simulink model "esercizio1_punto1"  (Simulink 7.6)
settings: Solver=ode45  StartTime=0.0  StopTime=10  MaxStep=.1  RelTol=1e-3  AbsTol=1e-3
values from neighbouring files (symbols this model uses):
  den = 1    [ASS1_SIS.M]    (also in ASS_APPR.M; ASS_SIS.M; MYFBODE.M = b; MYNYQ.M = b)
  den_appr = 1    [ASS_APPR.M]    (also in ASS_SIS.M)
  num = 0    [ASS1_SIS.M]    (also in ASS_SIS.M; MYFBODE.M = a; MYNYQ.M = a; nyquistnew.m = a)
  num_appr = 0    [ASS_APPR.M]
  T = 0    [ASS1_SIS.M]    (also in ASS_APPR.M = 0; end; ASS_SIS.M; MYFBODE.M = rit)
  T_appr = 0    [ASS_APPR.M]    (also in ASS_SIS.M = 0; end)
undefined symbols (not defined in the file or in its folder): ht, sfunyst, stt
settings Model: Creator=Ins  LastModifiedBy=Ins  ExtModeTrigMode=oneshot  ExtModeArmWhenConnect=off
settings DataIOCC: LimitDataPoints=off  SaveOutput=off  SaveTime=off  SignalLoggingName=sigsOut
settings OptimizationCC: BooleanDataType=off
settings DebuggingCC: SaveWithParameterizedLinksMsg=none  SignalResolutionControl=TryResolveAllWithWarning  SolverPrmCheckMsg=none  MultiTaskDSMMsg=warning  MultiTaskCondExecSysMsg=none  StrictBusMsg=None
settings HardwareCC: TargetUnknown=on
settings RTWCC: IncludeERTFirstTime=on

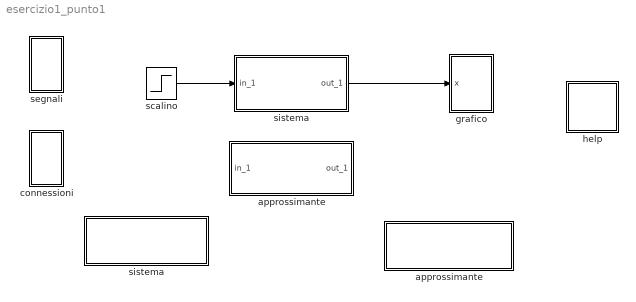
== system esercizio1_punto1 ==
  approssimante : Subsystem
      mask Display: disp('approssimante')
  "approssimante " : Subsystem
      settings: OpenFcn=blocca
      mask Display: disp('approssimante')
  connessioni : Subsystem
  grafico : Subsystem  mask(Storage scope.){npts =2000,  color ='b-/r-/c-./w:/m*/ro/b+'}
      mask prompts: npts  "Initial Time Range:";  color  "Initial y-min:"
      mask help:
      | Storage scope using MATLAB graph window.
      | Enter plotting ranges and line type.
      mask init:
      | ax = [0, @1, @2, @3]; dt=-1;
      mask Help: This block uses a MATLAB figure window to plot the input signal.  The graph limits are automatically scaled to the min and max values of the signal stored in the scope's signal buffer.  Line type must be in quotes.  See the M-file sfunyst.m.
      mask Display: plot(0,0,100,100,[83,76,63,52,42,38,28,16,11,84,11,11,11,90,90,11],[75,58,47,54,72,80,84,74,65,65,65,90,40,40,90,90])
  help : Subsystem
      mask Display: disp('?')
  scalino : Step  Time=0
  segnali : Subsystem
  sistema : Subsystem
      mask Display: disp('sistema')
  "sistema " : Subsystem
      settings: OpenFcn=blocca
      mask Display: disp('sistema')
  wires:
  "sistema "/1(out_1) -> grafico/1(x)
  scalino/1 -> "sistema "/1(in_1)

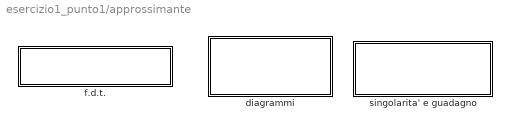
== system esercizio1_punto1/approssimante ==
  diagrammi : Subsystem
      mask Display: disp('diagrammi\n  \n (Bode e Nyquist)')
  f.d.t. : Subsystem
      settings: OpenFcn=ass_appr
      mask Type: assegnamento f.d.t.
      mask Display: disp('assegnamento f.d.t.')
  singolarita' e guadagno : Subsystem
      settings: OpenFcn=sing_app
      mask Type: singolarita' della f.d.t.
      mask Display: disp('singolarità,\n guadagno e ritardo')

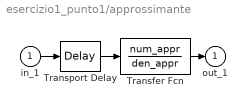
== system esercizio1_punto1/approssimante  ==
  in_1 : Inport
  Transfer Fcn : TransferFcn  Numerator=num_appr  Denominator=den_appr
  Transport Delay : TransportDelay  DelayTime=T_appr
  out_1 : Outport
  wires:
  Transport Delay/1 -> Transfer Fcn/1
  in_1/1 -> Transport Delay/1
  Transfer Fcn/1 -> out_1/1

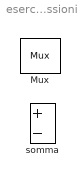
== system esercizio1_punto1/connessioni ==
  Mux : Mux  Inputs=2
  somma : Sum  Inputs=+-  SaturateOnIntegerOverflow=on  InputSameDT=on  OutDataTypeStr=Inherit: Same as first input

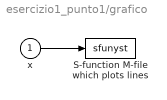
== system esercizio1_punto1/grafico ==
  x : Inport
  "S-function M-file which plots lines " : S-Function  LoadFcn=sfunyst([],[],[],'LoadBlock')  FunctionName=sfunyst  Parameters=ax, color, npts, dt  EnableBusSupport=off
      settings: CopyFcn=sfunyst([],[],[],'CopyBlock')  DeleteFcn=sfunyst([],[],[],'DeleteBlock')
  wires:
  x/1 -> "S-function M-file which plots lines "/1

== system esercizio1_punto1/help ==
  note: - il calcolo delle singolarità (poli e zeri), del guadagno e del ritardo della f.d.t.
  note: - l'inserimento della funzione di trasferimento
  note: - l'ottenimento dei diagrammi di Bode e di Nyquist
  note: i blocchi con l'ombreggiatura consentono

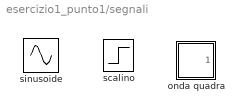
== system esercizio1_punto1/segnali ==
  onda quadra : Subsystem  mask(Pulse Generator){Ts=2,  du=1,  ht=1,  stt=0}
      mask prompts: Ts "Pulse period (secs):";  du "Pulse width:";  ht "Pulse height:";  stt "Pulse start time:"
      mask help: Pulse Generator.
      mask init:
      | ini=ones(length(ht),1); st1=rem(stt,Ts); st2=rem(stt+du,Ts);if(Ts<=1.2*du),ini=zeros(length(ht),1);end;
      mask Help: Pulse generator which ensures pulse\ntransitions are hit. Provides a vector of pulses when the height is entered as a vector.\nUnmask to see how it works.
      mask Display: plot(0,0,100,100,[90,75,75,60,60,35,35,20,20,10],[20,20,80,80,20,20,80,80,20,20])
  scalino : Step  Time=0
  sinusoide : Sin

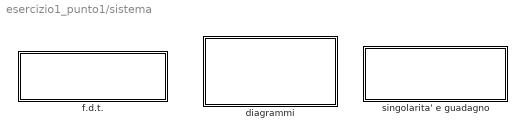
== system esercizio1_punto1/sistema ==
  diagrammi : Subsystem
      mask Display: disp('diagrammi\n  \n (Bode e Nyquist)')
  f.d.t. : Subsystem
      settings: OpenFcn=ass_sis
      mask Type: assegnamento f.d.t.
      mask Display: disp('assegnamento f.d.t.')
  singolarita' e guadagno : Subsystem
      settings: OpenFcn=sing_s
      mask Type: singolarita' della f.d.t.
      mask Display: disp('singolarità,\n guadagno e ritardo')

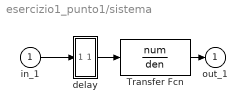
== system esercizio1_punto1/sistema  ==
  in_1 : Inport
  Transfer Fcn : TransferFcn  Numerator=num  Denominator=den
  delay : Subsystem
  out_1 : Outport
  wires:
  delay/1(out_1) -> Transfer Fcn/1
  in_1/1 -> delay/1(in_1)
  Transfer Fcn/1 -> out_1/1

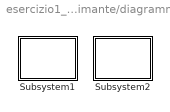
== system esercizio1_punto1/approssimante/diagrammi ==
  Subsystem1 : Subsystem
      settings: OpenFcn=nyq_appr
      mask Display: disp('Nyquist')
  Subsystem2 : Subsystem
      settings: OpenFcn=bode_app
      mask Display: disp('Bode')

== system esercizio1_punto1/approssimante/f.d.t. ==
  note: assegna

== system esercizio1_punto1/approssimante/singolarita' e guadagno ==
  note: assegna

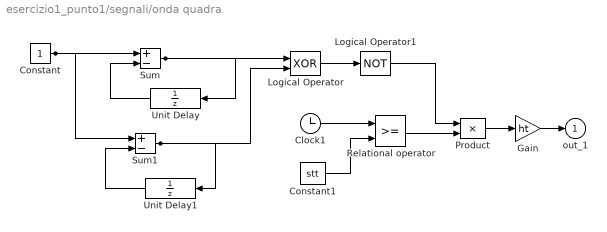
== system esercizio1_punto1/segnali/onda quadra ==
  Clock1 : Clock
      settings: Decimation=10
  Constant : Constant
  Constant1 : Constant  Value=stt
  Gain : Gain  Gain=ht  SaturateOnIntegerOverflow=on  OutDataTypeStr=Inherit: Same as input  ParamDataTypeStr=Inherit: Same as input
  Logical Operator : Logic  Operator=XOR
  Logical Operator1 : Logic  Operator=NOT  Inputs=1
  Product : Product  SaturateOnIntegerOverflow=on  InputSameDT=on  OutDataTypeStr=Inherit: Same as first input
  Relational operator : RelationalOperator  InputSameDT=on
  Sum : Sum  Inputs=+-  SaturateOnIntegerOverflow=on  InputSameDT=on  OutDataTypeStr=Inherit: Same as first input
  Sum1 : Sum  Inputs=+-  SaturateOnIntegerOverflow=on  InputSameDT=on  OutDataTypeStr=Inherit: Same as first input
  Unit Delay : UnitDelay  SampleTime=[Ts,st1]
  Unit Delay1 : UnitDelay  X0=ini  SampleTime=[Ts,st2]
  out_1 : Outport
  wires:
  Logical Operator1/1 -> Product/1
  Logical Operator/1 -> Logical Operator1/1
  Constant1/1 -> Relational operator/2
  Gain/1 -> out_1/1
  Product/1 -> Gain/1
  Relational operator/1 -> Product/2
  Clock1/1 -> Relational operator/1
  Unit Delay/1 -> Sum/2
  Unit Delay1/1 -> Sum1/2
  Constant/1 -> Sum/1, Sum1/1
  Sum/1 -> Unit Delay/1, Logical Operator/1
  Sum1/1 -> Unit Delay1/1, Logical Operator/2

== system esercizio1_punto1/sistema/diagrammi ==
  Bode : Subsystem
      settings: OpenFcn=bode_sis
      mask Display: disp('Bode')
  Nyquist : Subsystem
      settings: OpenFcn=nyq_sis
      mask Display: disp('Nyquist')

== system esercizio1_punto1/sistema/f.d.t. ==
  note: assegna

== system esercizio1_punto1/sistema/singolarita' e guadagno ==
  note: assegna

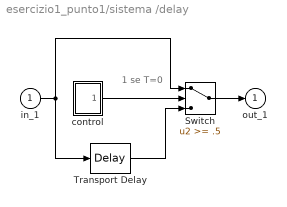
== system esercizio1_punto1/sistema /delay ==
  note: 1 se T=0
  in_1 : Inport
  Switch : Switch  Threshold=.5  SaturateOnIntegerOverflow=on  InputSameDT=on
  Transport Delay : TransportDelay  DelayTime=T
  control : Subsystem
  out_1 : Outport
  wires:
  Transport Delay/1 -> Switch/3
  in_1/1 -> Switch/1, Transport Delay/1
  Switch/1 -> out_1/1
  control/1(out_1) -> Switch/2

== system esercizio1_punto1/approssimante/diagrammi/Subsystem1 ==
  note: bode

== system esercizio1_punto1/approssimante/diagrammi/Subsystem2 ==
  note: bode

== system esercizio1_punto1/sistema/diagrammi/Bode ==
  note: bode

== system esercizio1_punto1/sistema/diagrammi/Nyquist ==
  note: nyquist

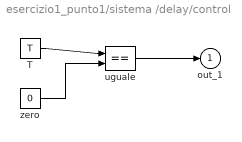
== system esercizio1_punto1/sistema /delay/control ==
  T : Constant  Value=T
  uguale : RelationalOperator  Operator===  InputSameDT=on
  zero : Constant  Value=0
  out_1 : Outport
  wires:
  zero/1 -> uguale/2
  T/1 -> uguale/1
  uguale/1 -> out_1/1
